simulink model "model"  (R2024a)
settings: Solver=VariableStepAuto  StartTime=0.0  StopTime=10.0  RelTol=1e-3
settings Model: Creator=eva  LastModifiedBy=eva

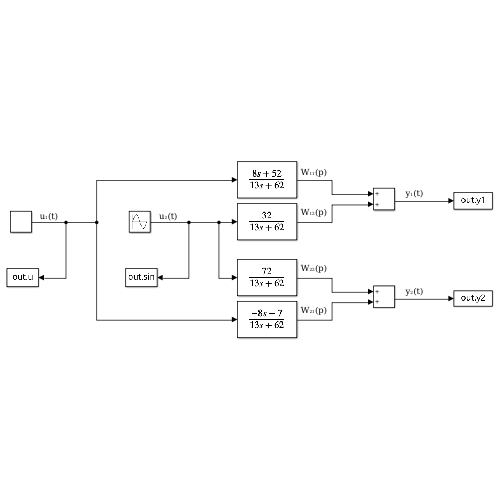
[thumbnail: Simulink's stored preview of the top-level diagram]
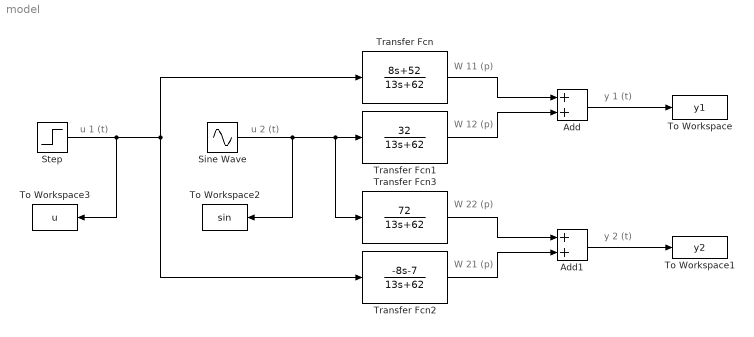
== system model ==
  note: u 1 (t)
  note: u 2 (t)
  note: W 11 (p)
  note: W 12 (p)
  note: W 22 (p)
  note: W 21 (p)
  note: y 2 (t)
  note: y 1 (t)
  Add : Sum
  Add1 : Sum
  Sine Wave : Sin  SampleTime=0
  Step : Step  Time=0  SampleTime=0
  To Workspace : ToWorkspace  VariableName=y1  SaveFormat=Structure With Time  SampleTime=-1
  To Workspace1 : ToWorkspace  VariableName=y2  SaveFormat=Structure With Time  SampleTime=-1
  To Workspace2 : ToWorkspace  VariableName=sin  SaveFormat=Structure With Time  SampleTime=-1
  To Workspace3 : ToWorkspace  VariableName=u  SaveFormat=Structure With Time  SampleTime=-1
  Transfer Fcn : TransferFcn  Numerator=[8 52]  Denominator=[13 62]
  Transfer Fcn1 : TransferFcn  Numerator=[32]  Denominator=[13 62]
  Transfer Fcn2 : TransferFcn  Numerator=[-8 -7]  Denominator=[13 62]
  Transfer Fcn3 : TransferFcn  Numerator=[72]  Denominator=[13 62]
  wires:
  Step/1 -> To Workspace3/1, Transfer Fcn2/1, Transfer Fcn/1
  Sine Wave/1 -> Transfer Fcn3/1, Transfer Fcn1/1, To Workspace2/1
  Transfer Fcn1/1 -> Add/2
  Add1/1 -> To Workspace1/1
  Transfer Fcn2/1 -> Add1/2
  Transfer Fcn3/1 -> Add1/1
  Transfer Fcn/1 -> Add/1
  Add/1 -> To Workspace/1
